simulink model "scars_example_stk"  (R2019b)
settings: Solver=ode14x  StartTime=0.0  StopTime=1.5*T  FixedStep=5  RelTol=1e-3
libraries: scars_library x2
settings Model: Creator=asmialek  LastModifiedBy=asmialek
settings DataIOCC: ReturnWorkspaceOutputsName=scars_out

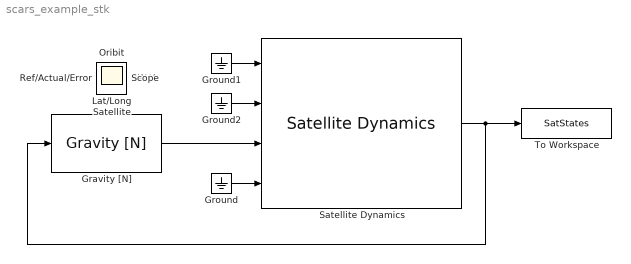
== system scars_example_stk ==
  Gravity [N] : scars_library/Environment/Gravity [N]  mass=1
  Ground : Ground
  Ground1 : Ground
  Ground2 : Ground
  Satellite Dynamics : scars_library/Advanced/Satellite Dynamics  Parameter4=LLA Position & NED Velocity, Rotation  epoch=2451545  mass=1  a=6371e3+400e3  e=0  incl=20  RA=0  w=0  TA=0  initEuler=[0 0 0]  initEulerRates=[0 0 90/120]  TA_copy=0  TA_copy_copy=400e3  TA_copy_copy_copy=[10 25]  TA_copy_copy_copy_copy=[1332.41761449570 7062.27056473502 -0.000303983477717348]  initEuler_copy=[0 0 0]  initEulerRates_copy=[0.01 0.02 0.005]  mask(Sattellite Dynamics){}
  To Workspace : ToWorkspace  VariableName=SatStates  SaveFormat=Timeseries  SampleTime=-1
  Lat/Long : Scope
  Oribit : Scope
  RW Y : Scope
  Ref/Actual/Error : Scope
  Satellite : Scope
  Scope : Scope
  wires:
  Ground/1 -> Satellite Dynamics/4
  Gravity [N]/1 -> Satellite Dynamics/3
  Ground1/1 -> Satellite Dynamics/1
  Ground2/1 -> Satellite Dynamics/2
  Satellite Dynamics/1 -> Gravity [N]/1, To Workspace/1
